simulink model "simulink_ALL"  (R2024b)
settings: Solver=FixedStepAuto  StartTime=0.0  StopTime=3000  FixedStep=10  RelTol=1e-3
values from neighbouring files (symbols this model uses):
  delay = 90    [MPC_utilizat.m]    (also in licenta.m)
  kd_ISE = kp_ISE*Td_ISE    (= 58.1981561553)    [licenta.m]
  kd_IST2E = kp_IST2E*Td_IST2E    (= 34.8986433055)    [licenta.m]
  kd_ISTE = kp_ISTE*Td_ISTE    (= 57.8649606048)    [licenta.m]
  ki_ISE = kp_ISE/Ti_ISE    (= 0.00295732865463)    [licenta.m]
  ki_IST2E = kp_IST2E/Ti_IST2E    (= 0.00228285218476)    [licenta.m]
  ki_ISTE = kp_ISTE/Ti_ISTE    (= 0.0023924364736)    [licenta.m]
  kp_ISE = Kp_ISE    (= 1.11283069815)    [licenta.m]
  kp_IST2E = Kp_IST2E    (= 1.03902553188)    [licenta.m]
  kp_ISTE = Kp_ISTE    (= 1.10645953003)    [licenta.m]
  kph = 2*420/(3*90*3.75)    (= 0.82962962963)    [licenta.m]
  kpl = tih/(kf*(lambda+delay))    [licenta.m]
  tih = 420    [MPC_utilizat.m]    (also in licenta.m)
libraries: cstblocks x41, mpclib x3
settings Model: Creator=Gabriel  LastModifiedBy=Gabriel

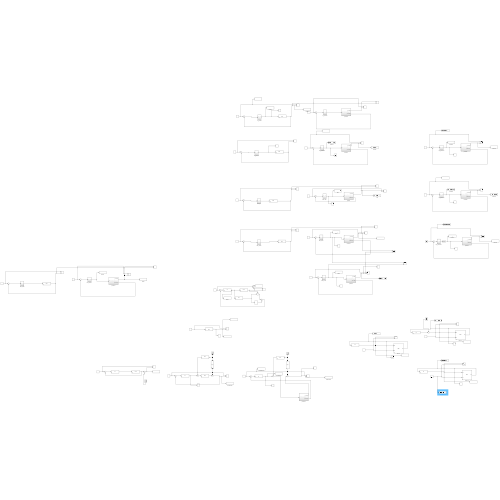
[thumbnail: Simulink's stored preview of the top-level diagram]
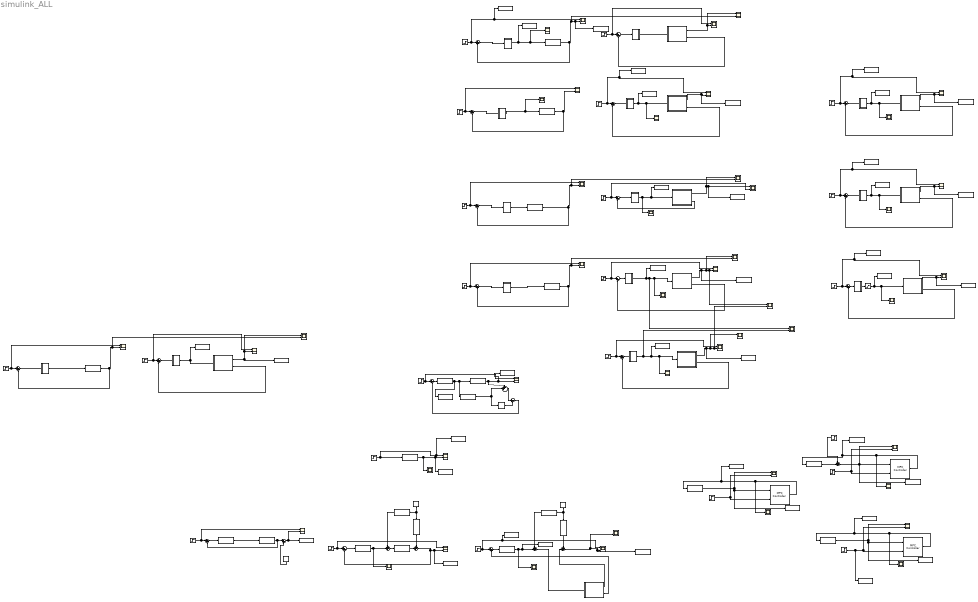
== system simulink_ALL ==
  Feedforward1 : ToWorkspace  VariableName=referinta_feedforward  SampleTime=-1
  Feedforward2 : ToWorkspace  VariableName=iesire_feedforward  SampleTime=-1
  Feedforward3 : ToWorkspace  VariableName=comanda_feedforward  SampleTime=-1
  Feedforward4 : ToWorkspace  VariableName=iesire_ff  SampleTime=-1
  ISE : ToWorkspace  VariableName=iesire_ISE  SampleTime=-1
  ISE1 : ToWorkspace  VariableName=comanda_ISE  SampleTime=-1
  IST2E : ToWorkspace  VariableName=iesire_IST2E  SampleTime=-1
  IST2E1 : ToWorkspace  VariableName=comanda_IST2E  SampleTime=-1
  ISTE1 : ToWorkspace  VariableName=comanda_ISTE  SampleTime=-1
  ISTE2 : ToWorkspace  VariableName=comanda_ISTE1  SampleTime=-1
  LTI System{1..3,19} (4 alike) : cstblocks/LTI System  sys=Gr  IC=[]  PadeOrder=0
  LTI System{6..7,9..12,22,42..43} (9 alike) : cstblocks/LTI System  sys=SYS  IC=[]  PadeOrder=0
  LTI System13 : cstblocks/LTI System  sys=hd  IC=[]  PadeOrder=0
  LTI System14 : cstblocks/LTI System  sys=hd  IC=[]  PadeOrder=0
  LTI System15 : cstblocks/LTI System  sys=hd  IC=[]  PadeOrder=0
  LTI System21 : cstblocks/LTI System  sys=Gff1  IC=[]  PadeOrder=0
  LTI System23 : cstblocks/LTI System  sys=Gp1  IC=[]  PadeOrder=0
  LTI System4 : cstblocks/LTI System  sys=Gff1  IC=[]  PadeOrder=0
  LTI System5 : cstblocks/LTI System  sys=Gp1  IC=[]  PadeOrder=0
  LTI System8 : cstblocks/LTI System  sys=Gm  IC=[]  PadeOrder=0
  Lambda : ToWorkspace  VariableName=iesire_Lambda  SampleTime=-1
  Lambda1 : ToWorkspace  VariableName=comanda_Lambda  SampleTime=-1
  MPC eu : mpclib/MPC Controller  SCDEnableBlockLinearizationSpecification=on  mpcobj=mpcobj  is_multiple=0  enable_value=0  return_u0=off  updateMPCinCallerWorkspace=on  md_inport=off  mv_inport=off  uref_inport=off  return_cost=off  return_mvseq=off  return_qpstatus=off  return_xseq=off  return_state=off  return_ovseq=off  state_inport=off  umin_inport=off  umax_inport=off  ymin_inport=off  ymax_inport=off  cc_inport=off  ywt_inport=off  uwt_inport=off  duwt_inport=off  rhoeps_inport=off  pm_inport=off  MaximumP=10  HorizonChoice=FixedHorizon  n_ts=10  n_p=120  n_mv=1  n_md=0  n_ud=0  n_mo=1  n_uo=0  BlockDataType=double  SampleTimeInherited=off  switch_inport=off
  MPC eu1 : mpclib/MPC Controller  SCDEnableBlockLinearizationSpecification=on  mpcobj=mpcobj  is_multiple=0  enable_value=0  return_u0=off  updateMPCinCallerWorkspace=on  md_inport=off  mv_inport=off  uref_inport=off  return_cost=off  return_mvseq=off  return_qpstatus=off  return_xseq=off  return_state=off  return_ovseq=off  state_inport=off  umin_inport=off  umax_inport=off  ymin_inport=off  ymax_inport=off  cc_inport=off  ywt_inport=off  uwt_inport=off  duwt_inport=off  rhoeps_inport=off  pm_inport=off  MaximumP=10  HorizonChoice=FixedHorizon  n_ts=10  n_p=120  n_mv=1  n_md=0  n_ud=0  n_mo=1  n_uo=0  BlockDataType=double  SampleTimeInherited=off  switch_inport=off
  MPC eu2 : mpclib/MPC Controller  SCDEnableBlockLinearizationSpecification=on  mpcobj=mpcobj  is_multiple=0  enable_value=0  return_u0=off  updateMPCinCallerWorkspace=on  md_inport=off  mv_inport=off  uref_inport=off  return_cost=off  return_mvseq=off  return_qpstatus=off  return_xseq=off  return_state=off  return_ovseq=off  state_inport=off  umin_inport=off  umax_inport=off  ymin_inport=off  ymax_inport=off  cc_inport=off  ywt_inport=off  uwt_inport=off  duwt_inport=off  rhoeps_inport=off  pm_inport=off  MaximumP=10  HorizonChoice=FixedHorizon  n_ts=10  n_p=120  n_mv=1  n_md=0  n_ud=0  n_mo=1  n_uo=0  BlockDataType=double  SampleTimeInherited=off  switch_inport=off
  REG_ISE : Subsystem
  REG_ISE1 : Subsystem
  REG_IST2E : Subsystem
  REG_IST2E1 : Subsystem
  REG_ISTE1 : Subsystem
  REG_ISTE2 : Subsystem
  REG_ISTE3 : Subsystem
  Random Number1 : RandomNumber
  Random Number2 : RandomNumber
  Random Number3 : RandomNumber
  Reg_Haalman : Subsystem
  Reg_Haalman1 : Subsystem
  Reg_Haalman2 : Subsystem
  Reg_Haalman3 : Subsystem
  Reg_Haalman4 : Subsystem
  Saturation : Saturate  UpperLimit=11  LowerLimit=0
  Scope{,2,11,13,22..24,27,31..32,34,36,38,40,43} (15 alike) : Scope
  Scope{1,3..10,12,14..21,25..26,28..30,33,35,37,39,41..42,44} (30 alike) : Scope  NumInputPorts=2
  Smith : ToWorkspace  VariableName=iesire_Smith  SampleTime=-1
  Smith1 : ToWorkspace  VariableName=comanda_Smith  SampleTime=-1
  Step{,1,3..5,7..11,13..18,23..24} (18 alike) : Step  Time=0  After=37
  Step12 : Step  Time=0  After=35
  Step19 : Step  Time=2000  Before=35  After=37
  Step2 : Step  Time=0  After=9
  Step20 : Step  Time=2000  After=-2
  Step6 : Step  Time=2000  Before=35  After=37
  Sum{,3,5,7,28..29} (6 alike) : Sum  Inputs=++|
  Sum{1..2,4,6,8..21,24} (19 alike) : Sum  Inputs=|+-
  Sum22 : Sum  Inputs=|++
  To Workspace : ToWorkspace  VariableName=referintalambda  SampleTime=-1
  To Workspace1 : ToWorkspace  VariableName=referinta_haalman  SampleTime=-1
  To Workspace10 : ToWorkspace  VariableName=referinta_haalman3  SampleTime=-1
  To Workspace11 : ToWorkspace  VariableName=iesire_MPC_eu1  SampleTime=-1
  To Workspace12 : ToWorkspace  VariableName=comanda_MPC_eu1  SampleTime=-1
  To Workspace13 : ToWorkspace  VariableName=iesire_MPC_eu2  SampleTime=-1
  To Workspace14 : ToWorkspace  VariableName=comanda_MPC_eu2  SampleTime=-1
  To Workspace15 : ToWorkspace  VariableName=iesire_poli  SampleTime=-1
  To Workspace16 : ToWorkspace  VariableName=ref_MPCs  SampleTime=-1
  To Workspace2 : ToWorkspace  VariableName=ref1  SampleTime=-1
  To Workspace3 : ToWorkspace  VariableName=com1  SampleTime=-1
  To Workspace4 : ToWorkspace  VariableName=iesire_ISTE1  SampleTime=-1
  To Workspace5 : ToWorkspace  VariableName=iesire_MPC_eu  SampleTime=-1
  To Workspace6 : ToWorkspace  VariableName=iesire_ISTE  SampleTime=-1
  To Workspace7 : ToWorkspace  VariableName=comanda_MPC_eu  SampleTime=-1
  To Workspace8 : ToWorkspace  VariableName=referinta_haalman1  SampleTime=-1
  To Workspace9 : ToWorkspace  VariableName=referinta_haalman2  SampleTime=-1
  Transport Delay1 : TransportDelay  DelayTime=delay
  haalman : ToWorkspace  VariableName=iesire_haalman  SampleTime=-1
  haalman1 : ToWorkspace  VariableName=comanda_haalman  SampleTime=-1
  haalman2 : ToWorkspace  VariableName=iesire_haalmanscref  SampleTime=-1
  haalman3 : ToWorkspace  VariableName=comanda_haalmanscref  SampleTime=-1
  haalman4 : ToWorkspace  VariableName=iesire_haalmanpert  SampleTime=-1
  haalman5 : ToWorkspace  VariableName=comanda_haalmanpert  SampleTime=-1
  haalman6 : ToWorkspace  VariableName=iesire_haalman11  SampleTime=-1
  haalman7 : ToWorkspace  VariableName=comanda_haalman11  SampleTime=-1
  predictor : Subsystem
  predictor1 : Subsystem
  predictor2 : Subsystem
  predictor3 : Subsystem
  predictor4 : Subsystem
  predictor5 : Subsystem
  predictor6 : Subsystem
  predictor7 : Subsystem
  predictor8 : Subsystem
  predictor9 : Subsystem
  reg_lambda : Subsystem
  reg_lambda1 : Subsystem
  wires:
  predictor4/1(y cu delay) -> Scope19/2, Scope20/1, IST2E/1
  Sum18/1 -> REG_IST2E1/1(In1)
  LTI System12/1 -> Sum19/2, Scope20/2, Scope21/2
  predictor4/2(y fara delay) -> Sum18/2
  REG_IST2E/1(Out1) -> LTI System12/1
  Sum19/1 -> REG_IST2E/1(In1)
  REG_IST2E1/1(u) -> predictor4/1(u), IST2E1/1
  Step14/1 -> Scope21/1, Sum19/1
  Step13/1 -> Scope19/1, Sum18/1
  Sum2/1 -> LTI System2/1
  LTI System6/1 -> Sum22/1, Sum2/2
  Step3/1 -> Scope3/1, Sum2/1
  LTI System2/1 -> LTI System6/1
  predictor3/1(y cu delay) -> To Workspace6/1, Scope17/1, Scope30/1, Scope16/2
  predictor3/2(y fara delay) -> Sum16/2
  Sum16/1 -> REG_ISTE1/1(In1)
  Step11/1 -> Scope16/1, Sum16/1
  LTI System11/1 -> Scope17/2, Scope18/2, Sum17/2
  Step12/1 -> Sum17/1, Scope18/1
  REG_ISTE2/1(Out1) -> LTI System11/1
  Sum17/1 -> REG_ISTE2/1(In1)
  Step9/1 -> Sum12/1, Scope9/1
  predictor/2(y fara delay) -> Sum10/2
  LTI System10/1 -> Scope8/2, Scope9/2, Sum12/2
  Sum10/1 -> REG_ISE1/1(In1)
  REG_ISE/1(Out1) -> LTI System10/1
  predictor/1(y cu delay) -> Scope8/1, ISE/1, Scope7/1
  Sum12/1 -> REG_ISE/1(In1)
  Step7/1 -> Scope7/2, Sum10/1
  REG_ISE1/1(Out1) -> Scope22/1, ISE1/1, predictor/1(u)
  predictor1/2(y fara delay) -> Sum11/2
  Reg_Haalman2/1(Out1) -> haalman1/1, Scope24/1, predictor1/1(u)
  Sum11/1 -> Reg_Haalman2/1(In1)
  LTI System42/1 -> Scope10/2, Sum13/2
  Sum13/1 -> Reg_Haalman/1(In1)
  Step23/1 -> Sum13/1, Scope10/1
  Reg_Haalman/1(Out1) -> Scope11/1, LTI System42/1
  predictor2/2(y fara delay) -> Sum14/2
  Step10/1 -> Sum15/1, To Workspace/1, Scope12/1
  Sum14/1 -> reg_lambda1/1(In1)
  reg_lambda1/1(Out1) -> predictor2/1(u)
  predictor2/1(y cu delay) -> Scope15/1, Scope14/2
  Step24/1 -> Scope14/1, Sum14/1
  Sum15/1 -> reg_lambda/1(In1)
  Sum5/1 -> Sum6/1
  Transport Delay1/1 -> Sum6/2
  LTI System8/1 -> Transport Delay1/1, Sum5/2
  Step4/1 -> Scope4/1, Sum4/1
  LTI System7/1 -> Smith/1, Scope4/2, Sum5/1
  Sum4/1 -> LTI System1/1
  Sum6/1 -> Sum4/2
  LTI System1/1 -> Smith1/1, LTI System8/1, LTI System7/1
  predictor5/1(y cu delay) -> Sum7/2
  LTI System21/1 -> Sum28/1
  Sum7/1 -> Scope5/2, Feedforward2/1, Scope1/2
  LTI System23/1 -> Sum29/1
  Sum24/1 -> LTI System19/1
  LTI System3/1 -> Sum3/2, Feedforward3/1, Scope2/1
  Random Number1/1 -> LTI System4/1, LTI System5/1
  Step1/1 -> Scope1/1, Feedforward1/1, Sum1/1
  predictor5/2(y fara delay) -> Sum1/2
  LTI System4/1 -> Sum3/1
  Step17/1 -> Scope28/1, Sum24/1
  Sum3/1 -> predictor5/1(u)
  Sum1/1 -> LTI System3/1
  Sum28/1 -> LTI System22/1
  LTI System5/1 -> Sum7/1
  Random Number2/1 -> LTI System21/1, LTI System23/1
  LTI System22/1 -> Sum29/2
  LTI System9/1 -> Scope/1, To Workspace2/1, Scope6/2
  Step2/1 -> To Workspace3/1, Scope6/1, LTI System9/1
  LTI System43/1 -> Scope15/2, Lambda/1, Scope12/2, Sum15/2
  reg_lambda/1(Out1) -> Lambda1/1, Scope13/1, LTI System43/1
  Step8/1 -> Scope42/1, To Workspace1/1, Sum11/1
  predictor1/1(y cu delay) -> haalman/1, Scope42/2
  REG_ISTE1/1(Out1) -> ISTE1/1, Scope29/1, Scope23/1, predictor3/1(u)
  REG_ISTE3/1(Out1) -> predictor6/1(u), Scope27/1, ISTE2/1, Scope29/2
  Step5/1 -> Sum8/1, Scope25/1
  Sum8/1 -> REG_ISTE3/1(In1)
  predictor6/2(y fara delay) -> Sum8/2
  predictor6/1(y cu delay) -> Scope30/2, Scope25/2, Scope26/1, To Workspace4/1
  LTI System19/1 -> Scope31/1, Sum28/2
  MPC eu/1 -> Scope32/1, To Workspace7/1, LTI System13/1
  Step/1 -> MPC eu/2, Scope33/2
  LTI System13/1 -> To Workspace5/1, MPC eu/1, Scope33/1
  predictor7/1(y cu delay) -> Scope35/2, haalman2/1
  Step6/1 -> Sum9/1, To Workspace8/1, Scope35/1
  Sum9/1 -> Reg_Haalman1/1(In1)
  Reg_Haalman1/1(Out1) -> predictor7/1(u), Scope34/1, haalman3/1
  predictor7/2(y fara delay) -> Sum9/2
  predictor8/2(y fara delay) -> Sum20/2
  Reg_Haalman3/1(Out1) -> haalman5/1, Scope36/1, predictor8/1(u)
  Sum20/1 -> Reg_Haalman3/1(In1)
  Step15/1 -> Scope37/1, To Workspace9/1, Sum20/1
  predictor8/1(y cu delay) -> haalman4/1, Scope37/2
  predictor9/1(y cu delay) -> Scope39/2, haalman6/1
  Step16/1 -> Sum21/1, To Workspace10/1, Scope39/1
  Sum21/1 -> Reg_Haalman4/1(In1)
  Reg_Haalman4/1(Out1) -> Saturation/1
  predictor9/2(y fara delay) -> Sum21/2
  Saturation/1 -> predictor9/1(u), Scope38/1, haalman7/1
  Step18/1 -> Scope41/2, MPC eu1/2
  MPC eu1/1 -> LTI System14/1, To Workspace12/1, Scope40/1
  MPC eu2/1 -> Scope43/1, To Workspace14/1, LTI System15/1
  Step19/1 -> To Workspace16/1, MPC eu2/2, Scope44/2
  LTI System15/1 -> To Workspace13/1, MPC eu2/1, Scope44/1
  Step20/1 -> Sum/1
  Sum/1 -> To Workspace11/1, Scope41/1, MPC eu1/1
  LTI System14/1 -> Sum/2
  Sum29/1 -> Feedforward4/1, Scope28/2, Sum24/2
  Random Number3/1 -> Sum22/2
  Sum22/1 -> Scope3/2, To Workspace15/1

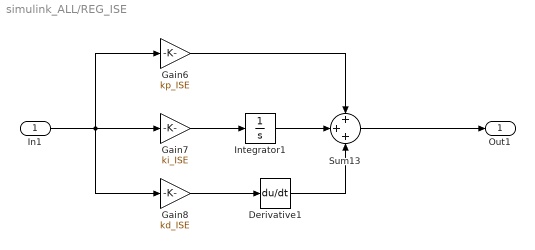
== system simulink_ALL/REG_ISE ==
  In1 : Inport
  Derivative1 : Derivative
  Gain6 : Gain  Gain=kp_ISE
  Gain7 : Gain  Gain=ki_ISE
  Gain8 : Gain  Gain=kd_ISE
  Integrator1 : Integrator
  Sum13 : Sum  Inputs=+++
  Out1 : Outport
  wires:
  In1/1 -> Gain8/1, Gain7/1, Gain6/1
  Gain7/1 -> Integrator1/1
  Gain6/1 -> Sum13/1
  Integrator1/1 -> Sum13/2
  Derivative1/1 -> Sum13/3
  Gain8/1 -> Derivative1/1
  Sum13/1 -> Out1/1

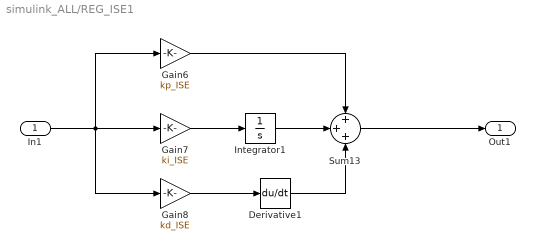
== system simulink_ALL/REG_ISE1 ==
  In1 : Inport
  Derivative1 : Derivative
  Gain6 : Gain  Gain=kp_ISE
  Gain7 : Gain  Gain=ki_ISE
  Gain8 : Gain  Gain=kd_ISE
  Integrator1 : Integrator
  Sum13 : Sum  Inputs=+++
  Out1 : Outport
  wires:
  In1/1 -> Gain8/1, Gain7/1, Gain6/1
  Gain7/1 -> Integrator1/1
  Gain6/1 -> Sum13/1
  Integrator1/1 -> Sum13/2
  Derivative1/1 -> Sum13/3
  Gain8/1 -> Derivative1/1
  Sum13/1 -> Out1/1

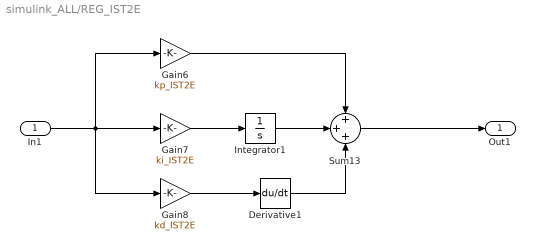
== system simulink_ALL/REG_IST2E ==
  In1 : Inport
  Derivative1 : Derivative
  Gain6 : Gain  Gain=kp_IST2E
  Gain7 : Gain  Gain=ki_IST2E
  Gain8 : Gain  Gain=kd_IST2E
  Integrator1 : Integrator
  Sum13 : Sum  Inputs=+++
  Out1 : Outport
  wires:
  Sum13/1 -> Out1/1
  Gain8/1 -> Derivative1/1
  Derivative1/1 -> Sum13/3
  Integrator1/1 -> Sum13/2
  Gain6/1 -> Sum13/1
  Gain7/1 -> Integrator1/1
  In1/1 -> Gain6/1, Gain7/1, Gain8/1

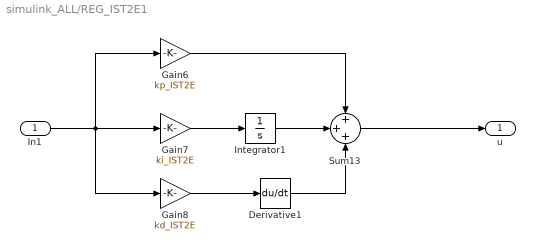
== system simulink_ALL/REG_IST2E1 ==
  In1 : Inport
  Derivative1 : Derivative
  Gain6 : Gain  Gain=kp_IST2E
  Gain7 : Gain  Gain=ki_IST2E
  Gain8 : Gain  Gain=kd_IST2E
  Integrator1 : Integrator
  Sum13 : Sum  Inputs=+++
  u : Outport
  wires:
  In1/1 -> Gain8/1, Gain7/1, Gain6/1
  Gain7/1 -> Integrator1/1
  Gain6/1 -> Sum13/1
  Integrator1/1 -> Sum13/2
  Derivative1/1 -> Sum13/3
  Gain8/1 -> Derivative1/1
  Sum13/1 -> u/1

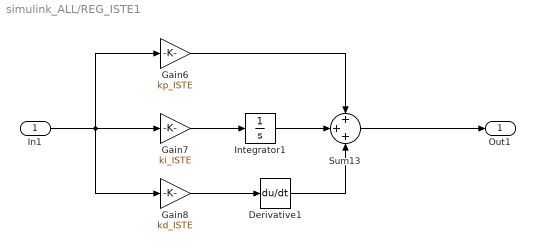
== system simulink_ALL/REG_ISTE1 ==
  In1 : Inport
  Derivative1 : Derivative
  Gain6 : Gain  Gain=kp_ISTE
  Gain7 : Gain  Gain=ki_ISTE
  Gain8 : Gain  Gain=kd_ISTE
  Integrator1 : Integrator
  Sum13 : Sum  Inputs=+++
  Out1 : Outport
  wires:
  Sum13/1 -> Out1/1
  Gain8/1 -> Derivative1/1
  Derivative1/1 -> Sum13/3
  Integrator1/1 -> Sum13/2
  Gain6/1 -> Sum13/1
  Gain7/1 -> Integrator1/1
  In1/1 -> Gain6/1, Gain7/1, Gain8/1

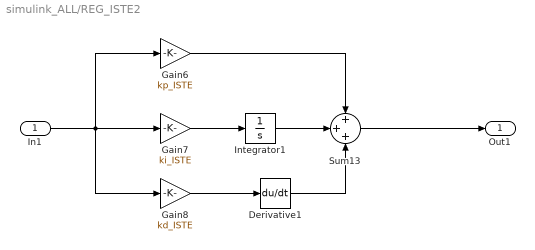
== system simulink_ALL/REG_ISTE2 ==
  In1 : Inport
  Derivative1 : Derivative
  Gain6 : Gain  Gain=kp_ISTE
  Gain7 : Gain  Gain=ki_ISTE
  Gain8 : Gain  Gain=kd_ISTE
  Integrator1 : Integrator
  Sum13 : Sum  Inputs=+++
  Out1 : Outport
  wires:
  In1/1 -> Gain8/1, Gain7/1, Gain6/1
  Gain7/1 -> Integrator1/1
  Gain6/1 -> Sum13/1
  Integrator1/1 -> Sum13/2
  Derivative1/1 -> Sum13/3
  Gain8/1 -> Derivative1/1
  Sum13/1 -> Out1/1

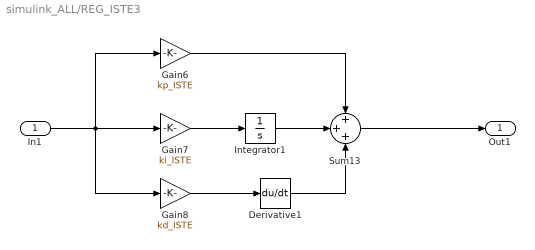
== system simulink_ALL/REG_ISTE3 ==
  In1 : Inport
  Derivative1 : Derivative
  Gain6 : Gain  Gain=kp_ISTE
  Gain7 : Gain  Gain=ki_ISTE
  Gain8 : Gain  Gain=kd_ISTE
  Integrator1 : Integrator
  Sum13 : Sum  Inputs=+++
  Out1 : Outport
  wires:
  In1/1 -> Gain8/1, Gain7/1, Gain6/1
  Gain7/1 -> Integrator1/1
  Gain6/1 -> Sum13/1
  Integrator1/1 -> Sum13/2
  Derivative1/1 -> Sum13/3
  Gain8/1 -> Derivative1/1
  Sum13/1 -> Out1/1

== system simulink_ALL/Reg_Haalman ==
  In1 : Inport
  Gain6 : Gain  Gain=kph
  Gain7 : Gain  Gain=kph/tih
  Integrator1 : Integrator
  Sum13 : Sum
  Out1 : Outport
  wires:
  In1/1 -> Gain7/1, Gain6/1
  Gain7/1 -> Integrator1/1
  Gain6/1 -> Sum13/1
  Integrator1/1 -> Sum13/2
  Sum13/1 -> Out1/1

== system simulink_ALL/Reg_Haalman1 ==
  In1 : Inport
  Gain6 : Gain  Gain=kph
  Gain7 : Gain  Gain=kph/tih
  Integrator1 : Integrator
  Sum13 : Sum
  Out1 : Outport
  wires:
  Sum13/1 -> Out1/1
  Integrator1/1 -> Sum13/2
  Gain6/1 -> Sum13/1
  Gain7/1 -> Integrator1/1
  In1/1 -> Gain6/1, Gain7/1

== system simulink_ALL/Reg_Haalman2 ==
  In1 : Inport
  Gain6 : Gain  Gain=kph
  Gain7 : Gain  Gain=kph/tih
  Integrator1 : Integrator
  Sum13 : Sum
  Out1 : Outport
  wires:
  In1/1 -> Gain7/1, Gain6/1
  Gain7/1 -> Integrator1/1
  Gain6/1 -> Sum13/1
  Integrator1/1 -> Sum13/2
  Sum13/1 -> Out1/1

== system simulink_ALL/Reg_Haalman3 ==
  In1 : Inport
  Gain6 : Gain  Gain=kph
  Gain7 : Gain  Gain=kph/tih
  Integrator1 : Integrator
  Sum13 : Sum
  Out1 : Outport
  wires:
  In1/1 -> Gain7/1, Gain6/1
  Gain7/1 -> Integrator1/1
  Gain6/1 -> Sum13/1
  Integrator1/1 -> Sum13/2
  Sum13/1 -> Out1/1

== system simulink_ALL/Reg_Haalman4 ==
  In1 : Inport
  Gain6 : Gain  Gain=kph
  Gain7 : Gain  Gain=kph/tih
  Integrator1 : Integrator
  Sum13 : Sum
  Out1 : Outport
  wires:
  Sum13/1 -> Out1/1
  Integrator1/1 -> Sum13/2
  Gain6/1 -> Sum13/1
  Gain7/1 -> Integrator1/1
  In1/1 -> Gain6/1, Gain7/1

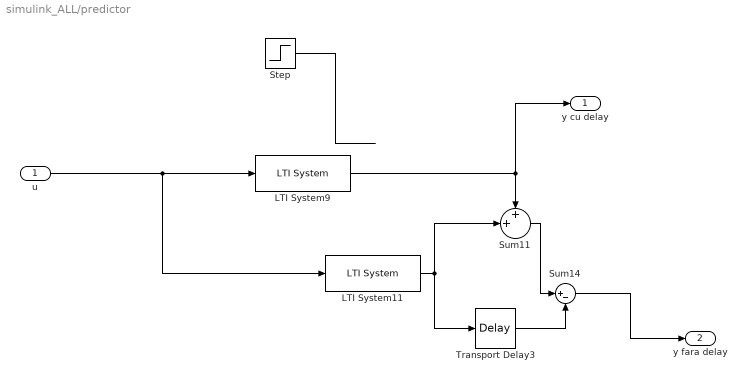
== system simulink_ALL/predictor ==
  u : Inport
  LTI System11 : cstblocks/LTI System  sys=Gm  IC=[]  PadeOrder=0
  LTI System9 : cstblocks/LTI System  sys=SYS  IC=[]  PadeOrder=0
  Step : Step  Time=2500  After=-5  SampleTime=0
  Sum11 : Sum  Inputs=++|
  Sum14 : Sum  Inputs=|+-
  Transport Delay3 : TransportDelay  DelayTime=delay
  y cu delay : Outport
  y fara delay : Outport  Port=2
  wires:
  u/1 -> LTI System9/1, LTI System11/1
  Sum11/1 -> Sum14/1
  LTI System11/1 -> Transport Delay3/1, Sum11/2
  Transport Delay3/1 -> Sum14/2
  Sum14/1 -> y fara delay/1
  Step/1 -> ?
  LTI System9/1 -> y cu delay/1, Sum11/1

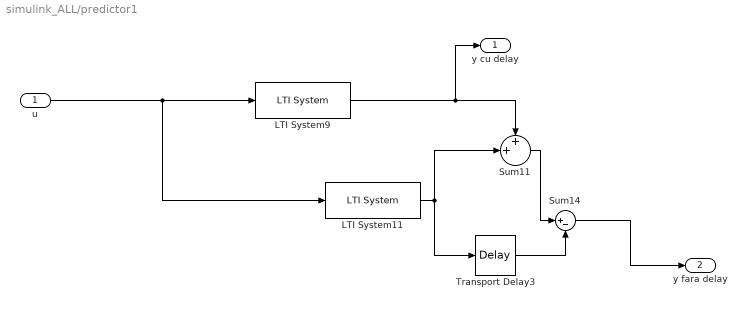
== system simulink_ALL/predictor1 ==
  u : Inport
  LTI System11 : cstblocks/LTI System  sys=Gm  IC=[]  PadeOrder=0
  LTI System9 : cstblocks/LTI System  sys=SYS  IC=[]  PadeOrder=0
  Sum11 : Sum  Inputs=++|
  Sum14 : Sum  Inputs=|+-
  Transport Delay3 : TransportDelay  DelayTime=delay
  y cu delay : Outport
  y fara delay : Outport  Port=2
  wires:
  u/1 -> LTI System9/1, LTI System11/1
  Sum11/1 -> Sum14/1
  LTI System11/1 -> Transport Delay3/1, Sum11/2
  Transport Delay3/1 -> Sum14/2
  LTI System9/1 -> y cu delay/1, Sum11/1
  Sum14/1 -> y fara delay/1

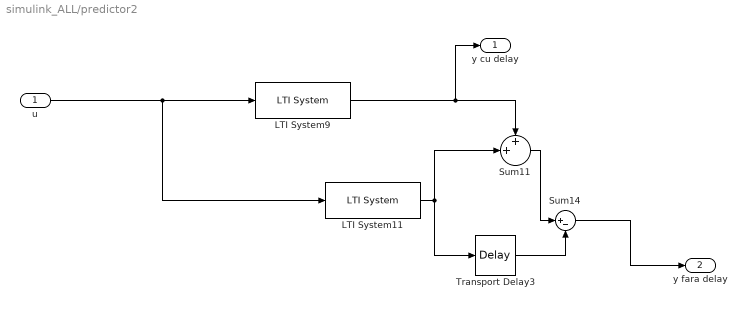
== system simulink_ALL/predictor2 ==
  u : Inport
  LTI System11 : cstblocks/LTI System  sys=Gm  IC=[]  PadeOrder=0
  LTI System9 : cstblocks/LTI System  sys=SYS  IC=[]  PadeOrder=0
  Sum11 : Sum  Inputs=++|
  Sum14 : Sum  Inputs=|+-
  Transport Delay3 : TransportDelay  DelayTime=delay
  y cu delay : Outport
  y fara delay : Outport  Port=2
  wires:
  u/1 -> LTI System9/1, LTI System11/1
  Sum11/1 -> Sum14/1
  LTI System11/1 -> Transport Delay3/1, Sum11/2
  Transport Delay3/1 -> Sum14/2
  LTI System9/1 -> y cu delay/1, Sum11/1
  Sum14/1 -> y fara delay/1

== system simulink_ALL/predictor3 ==
  u : Inport
  LTI System11 : cstblocks/LTI System  sys=Gm  IC=[]  PadeOrder=0
  LTI System9 : cstblocks/LTI System  sys=SYS  IC=[]  PadeOrder=0
  Sum11 : Sum  Inputs=++|
  Sum14 : Sum  Inputs=|+-
  Transport Delay3 : TransportDelay  DelayTime=delay
  y cu delay : Outport
  y fara delay : Outport  Port=2
  wires:
  u/1 -> LTI System9/1, LTI System11/1
  Sum11/1 -> Sum14/1
  LTI System11/1 -> Transport Delay3/1, Sum11/2
  Transport Delay3/1 -> Sum14/2
  LTI System9/1 -> y cu delay/1, Sum11/1
  Sum14/1 -> y fara delay/1

== system simulink_ALL/predictor4 ==
  u : Inport
  LTI System11 : cstblocks/LTI System  sys=Gm  IC=[]  PadeOrder=0
  LTI System9 : cstblocks/LTI System  sys=SYS  IC=[]  PadeOrder=0
  Sum11 : Sum  Inputs=++|
  Sum14 : Sum  Inputs=|+-
  Transport Delay3 : TransportDelay  DelayTime=delay
  y cu delay : Outport
  y fara delay : Outport  Port=2
  wires:
  Sum14/1 -> y fara delay/1
  LTI System9/1 -> Sum11/1, y cu delay/1
  Transport Delay3/1 -> Sum14/2
  LTI System11/1 -> Sum11/2, Transport Delay3/1
  Sum11/1 -> Sum14/1
  u/1 -> LTI System11/1, LTI System9/1

== system simulink_ALL/predictor5 ==
  u : Inport
  LTI System11 : cstblocks/LTI System  sys=Gm  IC=[]  PadeOrder=0
  LTI System9 : cstblocks/LTI System  sys=SYS  IC=[]  PadeOrder=0
  Sum11 : Sum  Inputs=++|
  Sum14 : Sum  Inputs=|+-
  Transport Delay3 : TransportDelay  DelayTime=delay
  y cu delay : Outport
  y fara delay : Outport  Port=2
  wires:
  u/1 -> LTI System9/1, LTI System11/1
  Sum11/1 -> Sum14/1
  LTI System11/1 -> Transport Delay3/1, Sum11/2
  Transport Delay3/1 -> Sum14/2
  LTI System9/1 -> y cu delay/1, Sum11/1
  Sum14/1 -> y fara delay/1

== system simulink_ALL/predictor6 ==
  u : Inport
  LTI System11 : cstblocks/LTI System  sys=Gm  IC=[]  PadeOrder=0
  LTI System9 : cstblocks/LTI System  sys=SYS  IC=[]  PadeOrder=0
  Sum11 : Sum  Inputs=++|
  Sum14 : Sum  Inputs=|+-
  Transport Delay3 : TransportDelay  DelayTime=delay
  y cu delay : Outport
  y fara delay : Outport  Port=2
  wires:
  Sum14/1 -> y fara delay/1
  LTI System9/1 -> Sum11/1, y cu delay/1
  Transport Delay3/1 -> Sum14/2
  LTI System11/1 -> Sum11/2, Transport Delay3/1
  Sum11/1 -> Sum14/1
  u/1 -> LTI System11/1, LTI System9/1

== system simulink_ALL/predictor7 ==
  u : Inport
  LTI System11 : cstblocks/LTI System  sys=Gm  IC=[]  PadeOrder=0
  LTI System9 : cstblocks/LTI System  sys=SYS  IC=[]  PadeOrder=0
  Sum11 : Sum  Inputs=++|
  Sum14 : Sum  Inputs=|+-
  Transport Delay3 : TransportDelay  DelayTime=delay
  y cu delay : Outport
  y fara delay : Outport  Port=2
  wires:
  Sum14/1 -> y fara delay/1
  LTI System9/1 -> Sum11/1, y cu delay/1
  Transport Delay3/1 -> Sum14/2
  LTI System11/1 -> Sum11/2, Transport Delay3/1
  Sum11/1 -> Sum14/1
  u/1 -> LTI System11/1, LTI System9/1

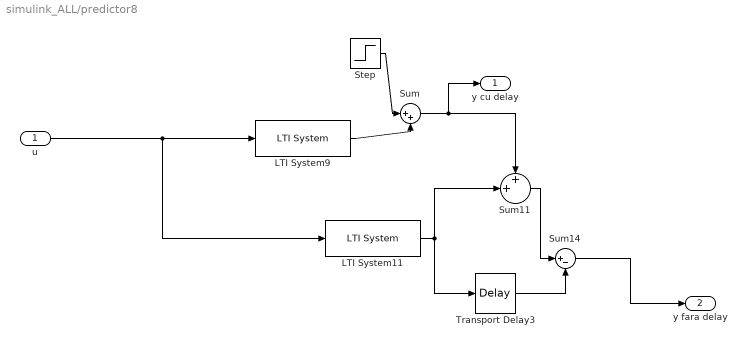
== system simulink_ALL/predictor8 ==
  u : Inport
  LTI System11 : cstblocks/LTI System  sys=Gm  IC=[]  PadeOrder=0
  LTI System9 : cstblocks/LTI System  sys=SYS  IC=[]  PadeOrder=0
  Step : Step  Time=2000  After=-2  SampleTime=0
  Sum : Sum  Inputs=|++
  Sum11 : Sum  Inputs=++|
  Sum14 : Sum  Inputs=|+-
  Transport Delay3 : TransportDelay  DelayTime=delay
  y cu delay : Outport
  y fara delay : Outport  Port=2
  wires:
  u/1 -> LTI System9/1, LTI System11/1
  Sum11/1 -> Sum14/1
  LTI System11/1 -> Transport Delay3/1, Sum11/2
  Transport Delay3/1 -> Sum14/2
  Sum14/1 -> y fara delay/1
  Step/1 -> Sum/1
  LTI System9/1 -> Sum/2
  Sum/1 -> y cu delay/1, Sum11/1

== system simulink_ALL/predictor9 ==
  u : Inport
  LTI System11 : cstblocks/LTI System  sys=Gm  IC=[]  PadeOrder=0
  LTI System9 : cstblocks/LTI System  sys=SYS  IC=[]  PadeOrder=0
  Sum11 : Sum  Inputs=++|
  Sum14 : Sum  Inputs=|+-
  Transport Delay3 : TransportDelay  DelayTime=delay
  y cu delay : Outport
  y fara delay : Outport  Port=2
  wires:
  LTI System9/1 -> Sum11/1, y cu delay/1
  Sum14/1 -> y fara delay/1
  Transport Delay3/1 -> Sum14/2
  LTI System11/1 -> Sum11/2, Transport Delay3/1
  Sum11/1 -> Sum14/1
  u/1 -> LTI System11/1, LTI System9/1

== system simulink_ALL/reg_lambda ==
  In1 : Inport
  Gain6 : Gain  Gain=kpl
  Gain7 : Gain  Gain=kpl/tih
  Integrator1 : Integrator
  Sum13 : Sum
  Out1 : Outport
  wires:
  In1/1 -> Gain7/1, Gain6/1
  Gain7/1 -> Integrator1/1
  Gain6/1 -> Sum13/1
  Integrator1/1 -> Sum13/2
  Sum13/1 -> Out1/1

== system simulink_ALL/reg_lambda1 ==
  In1 : Inport
  Gain6 : Gain  Gain=kph
  Gain7 : Gain  Gain=kpl/tih
  Integrator1 : Integrator
  Sum13 : Sum
  Out1 : Outport
  wires:
  In1/1 -> Gain7/1, Gain6/1
  Gain7/1 -> Integrator1/1
  Gain6/1 -> Sum13/1
  Integrator1/1 -> Sum13/2
  Sum13/1 -> Out1/1
